simulink library "light_sensor_calibration_algorithm_atomic_sub_chart_library"  (R2014b)
settings: Solver=ode45  StartTime=0.0  StopTime=10.0  RelTol=1e-3
libraries: legonxtlib x2
settings Model: Creator=mbiesiad  LastModifiedBy=pvinnako

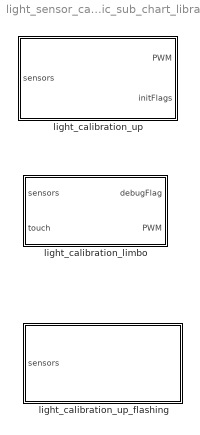
== system light_sensor_calibration_algorithm_atomic_sub_chart_library ==
  light_calibration_limbo : Stateflow chart  TreatAsAtomicUnit=on
  light_calibration_up : Stateflow chart  TreatAsAtomicUnit=on
  light_calibration_up_flashing : Stateflow chart  TreatAsAtomicUnit=on

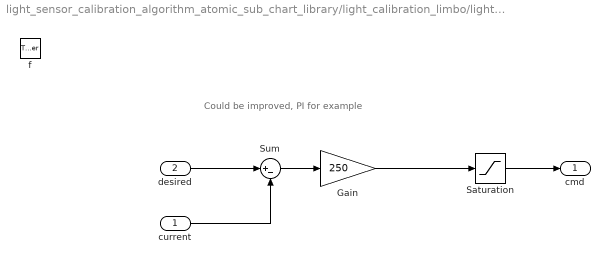
== system light_sensor_calibration_algorithm_atomic_sub_chart_library/light_calibration_limbo/light_sensor_calibration_limbo.tail_controller ==
  note: Could be improved, PI for example
  current : Inport  OutDataTypeStr=single  PortDimensions=1
  desired : Inport  Port=2  OutDataTypeStr=single  PortDimensions=1
  f : TriggerPort  TriggerType=function-call
      settings: CopyFcn=Stateflow.SLINSF.SimulinkMan.removeBlockPreDeleteFcn  PreDeleteFcn=Stateflow.SLINSF.SimulinkMan.unsafePredeleteFcn
  Gain : Gain  Gain=250
  Saturation : Saturate  UpperLimit=100  LowerLimit=-100  OutDataTypeStr=single
  Sum : Sum  Inputs=|+-
  cmd : Outport  OutDataTypeStr=single  PortDimensions=1  InitialOutput=0
  wires:
  Saturation/1 -> cmd/1
  Gain/1 -> Saturation/1
  desired/1 -> Sum/1
  current/1 -> Sum/2
  Sum/1 -> Gain/1

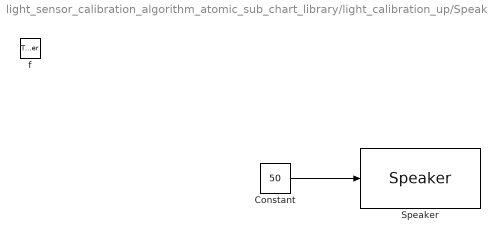
== system light_sensor_calibration_algorithm_atomic_sub_chart_library/light_calibration_up/Speak ==
  f : TriggerPort  TriggerType=function-call
      settings: CopyFcn=Stateflow.SLINSF.SimulinkMan.removeBlockPreDeleteFcn  PreDeleteFcn=Stateflow.SLINSF.SimulinkMan.unsafePredeleteFcn
  Constant : Constant  Value=50
  Speaker : legonxtlib/Speaker  sinputMode=Volume only  sspeakerFreq=800  sspeakerVolume=50  sspeakerDuration=100
  wires:
  Constant/1 -> Speaker/1

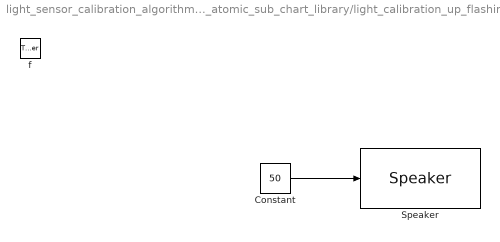
== system light_sensor_calibration_algorithm_atomic_sub_chart_library/light_calibration_up_flashing/LightSensorCalibFlashing.Speak ==
  f : TriggerPort  TriggerType=function-call
      settings: CopyFcn=Stateflow.SLINSF.SimulinkMan.removeBlockPreDeleteFcn  PreDeleteFcn=Stateflow.SLINSF.SimulinkMan.unsafePredeleteFcn
  Constant : Constant  Value=50
  Speaker : legonxtlib/Speaker  sinputMode=Volume only  sspeakerFreq=800  sspeakerVolume=50  sspeakerDuration=100
  wires:
  Constant/1 -> Speaker/1

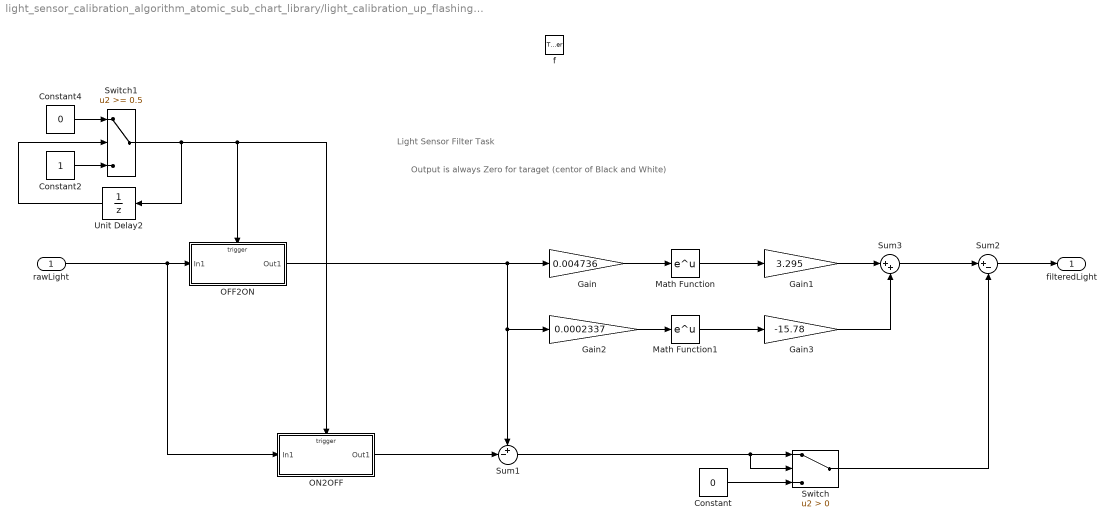
== system light_sensor_calibration_algorithm_atomic_sub_chart_library/light_calibration_up_flashing/LightSensorCalibFlashing.processLight ==
  note: Light Sensor Filter Task
  note: Output is always Zero for taraget (centor of Black and White)
  rawLight : Inport  OutDataTypeStr=single  PortDimensions=1
  f : TriggerPort  TriggerType=function-call
      settings: CopyFcn=Stateflow.SLINSF.SimulinkMan.removeBlockPreDeleteFcn  PreDeleteFcn=Stateflow.SLINSF.SimulinkMan.unsafePredeleteFcn
  Constant : Constant  Value=0  OutDataTypeStr=single  SampleTime=-1
  Constant2 : Constant  OutDataTypeStr=uint8
  Constant4 : Constant  Value=0  OutDataTypeStr=uint8
  Gain : Gain  Gain=0.004736
  Gain1 : Gain  Gain=3.295
  Gain2 : Gain  Gain=0.0002337
  Gain3 : Gain  Gain=-15.78
  Math Function : Math  SaturateOnIntegerOverflow=on
  Math Function1 : Math  SaturateOnIntegerOverflow=on
  OFF2ON : Subsystem  TreatAsAtomicUnit=on
  ON2OFF : Subsystem  TreatAsAtomicUnit=on
  Sum1 : Sum  Inputs=+-|
  Sum2 : Sum  Inputs=|+-
  Sum3 : Sum  Inputs=|++
  Switch : Switch  Criteria=u2 > Threshold  RndMeth=Simplest
  Switch1 : Switch  Threshold=0.5
  Unit Delay2 : UnitDelay  SampleTime=-1
  filteredLight : Outport  OutDataTypeStr=single  PortDimensions=1  InitialOutput=0
  wires:
  rawLight/1 -> OFF2ON/1(In1), ON2OFF/1(In1)
  Switch1/1 -> ON2OFF/Trigger, OFF2ON/Trigger, Unit Delay2/1
  Constant2/1 -> Switch1/3
  Constant4/1 -> Switch1/1
  Unit Delay2/1 -> Switch1/2
  ON2OFF/1(Out1) -> Sum1/2
  OFF2ON/1(Out1) -> Gain/1, Sum1/1, Gain2/1
  Gain/1 -> Math Function/1
  Math Function/1 -> Gain1/1
  Constant/1 -> Switch/3
  Sum1/1 -> Switch/1, Switch/2
  Gain2/1 -> Math Function1/1
  Math Function1/1 -> Gain3/1
  Gain1/1 -> Sum3/1
  Gain3/1 -> Sum3/2
  Sum3/1 -> Sum2/1
  Switch/1 -> Sum2/2
  Sum2/1 -> filteredLight/1

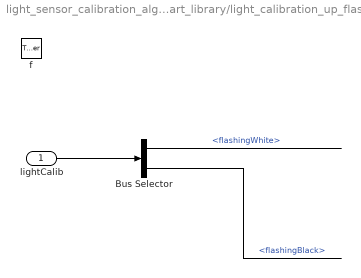
== system light_sensor_calibration_algorithm_atomic_sub_chart_library/light_calibration_up_flashing/LightSensorCalibFlashing.showCalib ==
  lightCalib : Inport  OutDataTypeStr=Bus: Light_Bus  PortDimensions=1
  f : TriggerPort  TriggerType=function-call
      settings: CopyFcn=Stateflow.SLINSF.SimulinkMan.removeBlockPreDeleteFcn  PreDeleteFcn=Stateflow.SLINSF.SimulinkMan.unsafePredeleteFcn
  Bus Selector : BusSelector  OutputSignals=flashingWhite,flashingBlack
  wires:
  Bus Selector/2 -> ?  "<flashingBlack>"
  Bus Selector/1 -> ?  "<flashingWhite>"
  lightCalib/1 -> Bus Selector/1

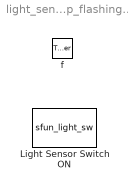
== system light_sensor_calibration_algorithm_atomic_sub_chart_library/light_calibration_up_flashing/LightSensorCalibFlashing.turnLightOn ==
  f : TriggerPort  TriggerType=function-call
      settings: CopyFcn=Stateflow.SLINSF.SimulinkMan.removeBlockPreDeleteFcn  PreDeleteFcn=Stateflow.SLINSF.SimulinkMan.unsafePredeleteFcn
  Light Sensor Switch ON : S-Function  FunctionName=sfun_light_sw  Parameters=-1,ip,sw  EnableBusSupport=off  mask(Light Sensor ON/OFF Switch){ip=S3, sw=ON}
      mask prompts: ip "port:"; sw "switch"
      mask help: LEGO Mindstorms NXT Light Sensor switch.
      mask init:
      | [data, map]=imread('LIGHT_SENSOR.gif');
      | pic=ind2rgb(data,map);
      mask TypeOptions ip: S1 | S2 | S3 | S4
      mask TypeOptions sw: ON | OFF
      mask Display:
      | image(pic)
      | color('red')
      | fprintf('%s, %s',ip,sw)

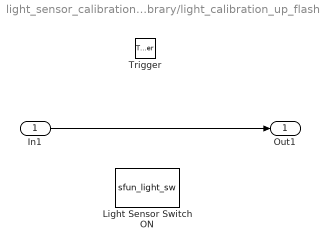
== system light_sensor_calibration_algorithm_atomic_sub_chart_library/light_calibration_up_flashing/LightSensorCalibFlashing.processLight/OFF2ON ==
  In1 : Inport
  Trigger : TriggerPort
  Light Sensor Switch ON : S-Function  FunctionName=sfun_light_sw  Parameters=-1,ip,sw  EnableBusSupport=off  mask(Light Sensor ON/OFF Switch){ip=S3, sw=ON}
      mask prompts: ip "port:"; sw "switch"
      mask help: LEGO Mindstorms NXT Light Sensor switch.
      mask init:
      | [data, map]=imread('LIGHT_SENSOR.gif');
      | pic=ind2rgb(data,map);
      mask TypeOptions ip: S1 | S2 | S3 | S4
      mask TypeOptions sw: ON | OFF
      mask Display:
      | image(pic)
      | color('red')
      | fprintf('%s, %s',ip,sw)
  Out1 : Outport
  wires:
  In1/1 -> Out1/1

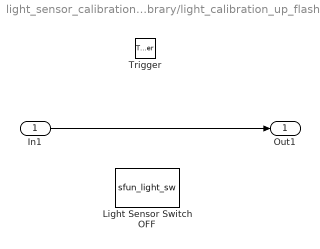
== system light_sensor_calibration_algorithm_atomic_sub_chart_library/light_calibration_up_flashing/LightSensorCalibFlashing.processLight/ON2OFF ==
  In1 : Inport
  Trigger : TriggerPort  TriggerType=falling
  Light Sensor Switch OFF : S-Function  FunctionName=sfun_light_sw  Parameters=-1,ip,sw  EnableBusSupport=off  mask(Light Sensor ON/OFF Switch){ip=S3, sw=OFF}
      mask prompts: ip "port:"; sw "switch"
      mask help: LEGO Mindstorms NXT Light Sensor switch.
      mask init:
      | [data, map]=imread('LIGHT_SENSOR.gif');
      | pic=ind2rgb(data,map);
      mask TypeOptions ip: S1 | S2 | S3 | S4
      mask TypeOptions sw: ON | OFF
      mask Display:
      | image(pic)
      | color('red')
      | fprintf('%s, %s',ip,sw)
  Out1 : Outport
  wires:
  In1/1 -> Out1/1

== stateflow chart light_sensor_calibration_algorithm_atomic_sub_chart_library/light_calibration_limbo ==
  state light_sensor_calibration_limbo
    entry:
    desired_tail = single(1.6);
    entry, during,exit:
    PWM.tail = tail_controller(sensors.theta_T,desired_tail);
    state TiltDown
      entry: debugFlag = uint16(409);
      during:
      desired_tail = desired_tail - single(0.3/(1/0.004));
    state WaitForBlack
      entry: debugFlag = uint16(410);
    state StoreBlackonTail
      entry: lightCalib.blackOnLimbo = sensors.light;
      debugFlag = uint16(sensors.light);
    state WaitForWhiteOnTail
      %entry: debugFlag = uint16(416)
    state StoreWhiteOnTail
      entry: lightCalib.whiteOnLimbo = sensors.light;
      debugFlag = uint16(sensors.light);
    state CalibComplete
      entry:
      %debugFlag = uint16(318);
      current_task_operation_status = OperationModeStatusEnum.SUCCESSFULLY_COMPLETED;
    state cmd = tail_controller(current,desired) [function]
    (default) -> TiltDown
    TiltDown -> WaitForBlack : [desired_tail <= 1.1]
    WaitForBlack -> StoreBlackonTail : [hasChangedFrom(touch,single(0))]
    StoreBlackonTail -> WaitForWhiteOnTail : after(1,sec)
    WaitForWhiteOnTail -> StoreWhiteOnTail : [hasChangedFrom(touch,single(0))]
    StoreWhiteOnTail -> CalibComplete : after(1,sec)
  data: current function_input single size=1; desired function_input single size=1; cmd function_output single size=1; sensors input Bus: Sensors_Bus size=1; lightCalib data_store_memory; current_task_operation_status data_store_memory; debugFlag output uint16; touch input single size=1; PWM output Bus: PWM_bus size=1; desired_tail local

== stateflow chart light_sensor_calibration_algorithm_atomic_sub_chart_library/light_calibration_up_flashing ==
  state LightSensorCalibFlashing
    during:
    on every(3, tick): filteredLight = processLight(sensors.light);
    % showCalib(lightCalib);
    state WaitForBlack
      entry: StatusLCD( uint16(310));
    state StoreBlack
      entry: lightCalib.flashingBlack = filteredLight;
      StatusLCD(uint16(311));
      Speak;
    state WaitForWhite
      entry:StatusLCD(uint16(312));
      Speak;
    state showCalib(lightCalib) [function] [commented out]
    state StoreWhite
      entry: lightCalib.flashingWhite = filteredLight;
      StatusLCD(uint16(313));
      Speak;
      exit:
      turnLightOn;
      Speak;
    state CalibComplete
      entry:
      StatusLCD(uint16(318));
      current_task_operation_status = OperationModeStatusEnum.SUCCESSFULLY_COMPLETED;
    state Speak [function] [commented out]
    state turnLightOn [function]
    state filteredLight  = processLight(rawLight) [function]
    (default) -> WaitForBlack
    WaitForBlack -> StoreBlack : [sensors.touch]{Speak;}
    StoreBlack -> WaitForWhite : after(1,sec)
    WaitForWhite -> StoreWhite : [sensors.touch]{Speak;}
    StoreWhite -> CalibComplete : after(1,sec)
  data: lightCalib function_input double; rawLight function_input single size=1; filteredLight function_output single size=1; sensors input Bus: Sensors_Bus size=1; lightCalib data_store_memory; current_task_operation_status data_store_memory; filteredLight local

== stateflow chart light_sensor_calibration_algorithm_atomic_sub_chart_library/light_calibration_up ==
  state wait
    entry: StatusLCD(uint16(200));
  state MoveUp
    entry: StatusLCD(uint16(201));
    PWM.tail = single(-50);
  state Reset
    entry:StatusLCD(uint16(202));
    PWM.tail = single(0);
    initFlags.tail = single(1);
    exit:
    initFlags.tail = single(0);
    desired_tail = single(0);
  state light_sensor_calibration_up
    %during, exit: PWM.tail = tail_controller(sensors.theta_T,single(1.6))
    state WaitForBlack
      entry: StatusLCD(uint16(310));
    state StoreBlack
      entry: lightCalib.black = sensors.light;
      StatusLCD(uint16(311));
    state WaitForWhite
      entry: StatusLCD(uint16(312));
    state StoreWhite
      entry: lightCalib.white = sensors.light;
      StatusLCD(uint16(313));
    state CalibComplete
      entry:
      StatusLCD(uint16(318));
      current_task_operation_status = OperationModeStatusEnum.SUCCESSFULLY_COMPLETED;
    (default) -> WaitForBlack
    WaitForBlack -> StoreBlack : [sensors.touch]{Speak;}
    StoreBlack -> WaitForWhite : after(0.2,sec){Speak;}
    WaitForWhite -> StoreWhite : [sensors.touch]{Speak;}
    StoreWhite -> CalibComplete : after(0.2,sec){Speak;}
  state Speak [function] [commented out]
  (default) -> wait
  wait -> MoveUp : [sensors.touch]{Speak;}
  MoveUp -> Reset : after(2,sec)
  Reset -> light_sensor_calibration_up : after(1,sec){Speak;}
  data: sensors input Bus: Sensors_Bus size=1; lightCalib data_store_memory; current_task_operation_status data_store_memory; PWM output Bus: PWM_bus size=1; initFlags output Bus: Init_Bus size=1; desired_tail local
